simulink model "rd3_mimo_sim_max"  (R2017b)
settings: Solver=ode23tb  StartTime=0.0  StopTime=tsim  FixedStep=0.001  RelTol=1e-3
values from neighbouring files (symbols this model uses):
  a20 = 1    [SISO_Example.m]
  a21 = 2    [SISO_Example.m]
  a22 = 1    [SISO_Example.m]
  Aa = [A,zeros(length(A),length(index_output)) ... (first row only)    [SimVFA.m]
  Aa_M = zeros([12,12,length(TP.etasweep)])    [SimVFA.m]
  Ba = [B; zeros(length(index_output),num_input)]    [SimVFA.m]
  Ba32_aug_M = zeros([12,3,length(TP.etasweep)])    [SimVFA.m]
  Ba32_M = zeros([12,2,length(TP.etasweep)])    [SimVFA.m]
  Ba3_aug_M = zeros([12,3,length(TP.etasweep)])    [SimVFA.m]
  Ba3_M = zeros([12,2,length(TP.etasweep)])    [SimVFA.m]
  Bp = B_c_hold(:,:,SO.eta_nom+1)    [SimVFA.m]
  Ca = [C, zeros(size(C,1),length(index_output)) ... (first row only)    [SimVFA.m]
  Cz = [0,0,0,0,1,0,0,0,0,0 ... (first row only)    [SimVFA.m]
  Kr_M = zeros([2,12,length(TP.etasweep)])    [SimVFA.m]
  Las = Uinv*Lis    [SimVFA.m]
  Las_M = zeros([12,3,length(TP.etasweep)])    [SimVFA.m]
  Ras_M = zeros([3,3,length(TP.etasweep)])    [SimVFA.m]
  Sas1_M = zeros([2,3,length(TP.etasweep)])    [SimVFA.m]
  Sas_M = zeros([3,3,length(TP.etasweep)])    [SimVFA.m]
undefined symbols (not defined in the file or in its folder): Aact, Acmd, Ada_Flag, ahold, Apsim, Bact, Bact_x, Bcmd, Bm, Cact, Cact_dot, Caz, Ccmd, Ccmd_dot, Cm, d00, d10, d11, d20, d21, d22, d_sam, data, Dz, Gamma_l, Gamma_p1, Gamma_p2, Gamma_p3, Gamma_p31, Gamma_p31xm, Gamma_p32, Gamma_vl, i_input_sel, i_state_sel, initstate, input_hold, inputselect, lambda_0, Lambda_s, mu_lambda, mu_psi1, mu_psi2, mu_psi3, mu_psi31, mu_psi32, n_sam, psi1_0, psi2_0, psi31_0, psi31xm_0, psi32_0, psi3_0, samplet, Si1, Si3, state_hold, vlambda_0, x_red_est_0
libraries: simulink x6
(part 1 of 2)
settings Model: SimulationMode=accelerator  Creator=Travis  LastModifiedBy=ben
settings DataIOCC: LimitDataPoints=on  SaveFormat=Structure  SignalLoggingSaveFormat=ModelDataLogs  SaveOutput=off  SignalLogging=off  DSMLogging=off  SaveTime=off  ReturnWorkspaceOutputs=on
settings OptimizationCC: BlockReduction=off  DefaultParameterBehavior=Inlined  BufferReuse=off  ExpressionDepthLimit=2147483647  InitFltsAndDblsToZero=on  LifeSpan=inf
settings DebuggingCC: SaveWithParameterizedLinksMsg=none  UnderspecifiedInitializationDetection=Classic  MergeDetectMultiDrivingBlocksExec=none  SignalResolutionControl=TryResolveAllWithWarning  SolverPrmCheckMsg=warning  MultiTaskDSMMsg=warning  MultiTaskCondExecSysMsg=none  FcnCallInpInsideContextMsg=warning  StateNameClashWarn=warning  StrictBusMsg=Warning  SFUnexpectedBacktrackingDiag=warning  SFNoUnconditionalDefaultTransitionDiag=warning  SFExecutionAtInitializationDiag=none
settings HardwareCC: ProdBitPerPointer=32  ProdBitPerSizeT=32  ProdBitPerPtrDiffT=32  ProdLargestAtomicFloat=None  ProdIntDivRoundTo=Undefined  ProdEndianess=Unspecified  ProdWordSize=32  ProdHWDeviceType=32-bit Generic
settings ModelReferenceCC: PropagateSignalLabelsOutOfModel=off
settings CodeAppCC: StateflowObjectComments=on
settings GRTTargetCC: TargetFcnLib=ansi_tfl_tmw.mat  TargetLangStandard=C89/C90 (ANSI)  GeneratePreprocessorConditionals=Disable all  CombineOutputUpdateFcns=off  GRTInterface=on
settings ConfigComp: CovMetricSettings=dw  CovHtmlReporting=on  CovSaveCumulativeToWorkspaceVar=on  CovSaveSingleToWorkspaceVar=on  CovExternalEMLEnable=off

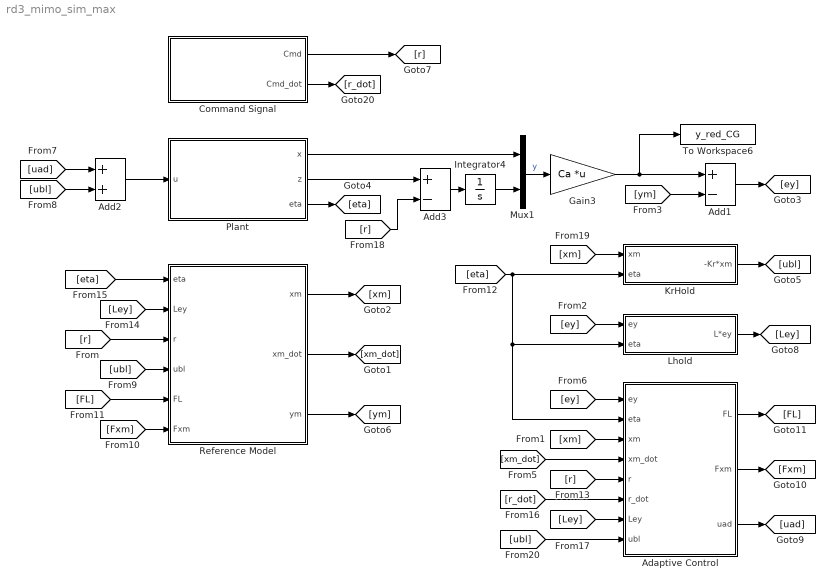
== system rd3_mimo_sim_max ==
  Adaptive Control : Subsystem
  Add1 : Sum  Inputs=+-
  Add2 : Sum
  Add3 : Sum  Inputs=+-
  Command Signal : Subsystem
  Gain3 : Gain  Gain=Ca  Multiplication=Matrix(K*u)
  Integrator4 : Integrator
  KrHold : Subsystem
  Lhold : Subsystem
  Mux1 : Mux  Inputs=2
  Plant : Subsystem
  Reference Model : Subsystem
  To Workspace6 : ToWorkspace  VariableName=y_red_CG  SampleTime=-1
      settings: Decimation=data_deci
  wires:
  Command Signal/1(Cmd) -> [r]
  [ey] -> Lhold/1(ey)
  Lhold/1(L*ey) -> [Ley]
  Mux1/1 -> Gain3/1  "y"
  Command Signal/2(Cmd_dot) -> [r_dot]
  [ym] -> Add1/2
  Add1/1 -> [ey]
  [uad] -> Add2/1
  [ubl] -> Add2/2
  [ey] -> Adaptive Control/1(ey)
  Adaptive Control/1(FL) -> [FL]
  Adaptive Control/2(Fxm) -> [Fxm]
  Adaptive Control/3(uad) -> [uad]
  [eta] -> Lhold/2(eta), Adaptive Control/2(eta), KrHold/2(eta)
  [eta] -> Reference Model/1(eta)
  [Ley] -> Reference Model/2(Ley)
  [r] -> Reference Model/3(r)
  [ubl] -> Reference Model/4(ubl)
  [FL] -> Reference Model/5(FL)
  [Fxm] -> Reference Model/6(Fxm)
  Reference Model/1(xm) -> [xm]
  Reference Model/2(xm_dot) -> [xm_dot]
  Integrator4/1 -> Mux1/2
  Add2/1 -> Plant/1(u)
  Plant/1(x) -> Mux1/1
  Add3/1 -> Integrator4/1
  Plant/2(z) -> Add3/1
  [r] -> Add3/2
  KrHold/1(-Kr*xm) -> [ubl]
  [xm] -> KrHold/1(xm)
  Reference Model/3(ym) -> [ym]
  Gain3/1 -> To Workspace6/1, Add1/1
  [xm] -> Adaptive Control/3(xm)
  [xm_dot] -> Adaptive Control/4(xm_dot)
  [r] -> Adaptive Control/5(r)
  [r_dot] -> Adaptive Control/6(r_dot)
  [Ley] -> Adaptive Control/7(Ley)
  [ubl] -> Adaptive Control/8(ubl)
  Plant/3(eta) -> [eta]

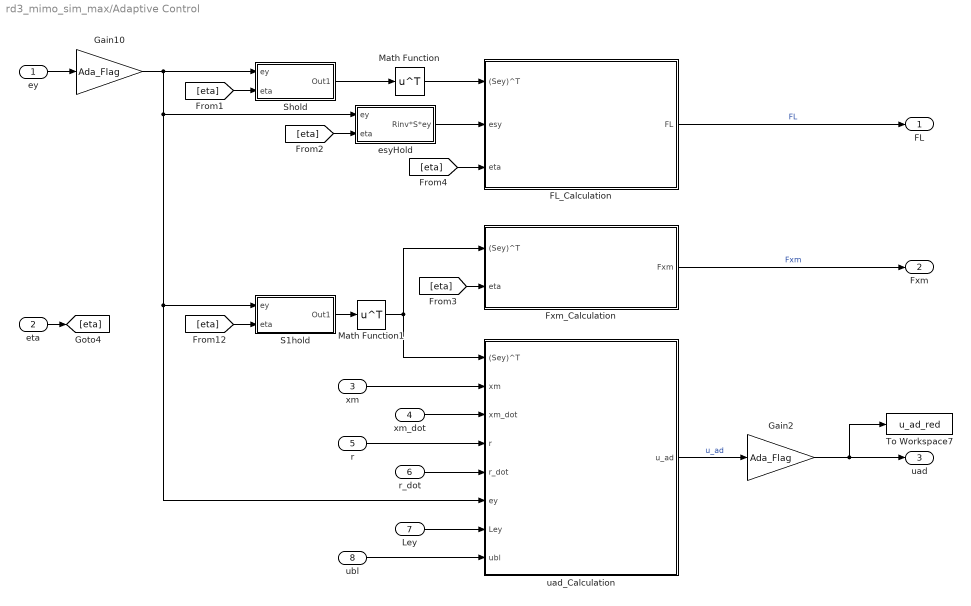
== system rd3_mimo_sim_max/Adaptive Control ==
  ey : Inport
  eta : Inport  Port=2
  xm : Inport  Port=3
  xm_dot : Inport  Port=4
  r : Inport  Port=5
  r_dot : Inport  Port=6
  Ley : Inport  Port=7
  ubl : Inport  Port=8
  FL_Calculation : Subsystem
  Fxm_Calculation : Subsystem
  Gain10 : Gain  Gain=Ada_Flag
  Gain2 : Gain  Gain=Ada_Flag
  Math Function : Math  Operator=transpose  SaturateOnIntegerOverflow=on
  Math Function1 : Math  Operator=transpose  SaturateOnIntegerOverflow=on
  S1hold : Subsystem
  Shold : Subsystem
  To Workspace7 : ToWorkspace  VariableName=u_ad_red  SampleTime=-1
      settings: Decimation=data_deci
  esyHold : Subsystem
  uad_Calculation : Subsystem
  FL : Outport
  Fxm : Outport  Port=2
  uad : Outport  Port=3
  wires:
  Shold/1(Out1) -> Math Function/1
  Math Function/1 -> FL_Calculation/1((Sey)^T)
  S1hold/1(Out1) -> Math Function1/1
  Math Function1/1 -> uad_Calculation/1((Sey)^T), Fxm_Calculation/1((Sey)^T)
  Gain10/1 -> Shold/1(ey), esyHold/1(ey), S1hold/1(ey), uad_Calculation/6(ey)
  uad_Calculation/1(u_ad) -> Gain2/1  "u_ad"
  ey/1 -> Gain10/1
  Fxm_Calculation/1(Fxm) -> Fxm/1  "Fxm"
  FL_Calculation/1(FL) -> FL/1  "FL"
  Gain2/1 -> To Workspace7/1, uad/1
  xm/1 -> uad_Calculation/2(xm)
  xm_dot/1 -> uad_Calculation/3(xm_dot)
  r/1 -> uad_Calculation/4(r)
  r_dot/1 -> uad_Calculation/5(r_dot)
  Ley/1 -> uad_Calculation/7(Ley)
  ubl/1 -> uad_Calculation/8(ubl)
  esyHold/1(Rinv*S*ey) -> FL_Calculation/2(esy)
  eta/1 -> [eta]
  [eta] -> S1hold/2(eta)
  [eta] -> Shold/2(eta)
  [eta] -> esyHold/2(eta)
  [eta] -> Fxm_Calculation/2(eta)
  [eta] -> FL_Calculation/3(eta)

== system rd3_mimo_sim_max/Command Signal ==
  Clock : Clock
  Filter : Subsystem
  From Workspace : FromWorkspace  VariableName=r_timeseries  SampleTime=0  Interpolate=off  OutputAfterFinalValue=Holding final value
  To Workspace14 : ToWorkspace  VariableName=r_cmd  SampleTime=-1
      settings: Decimation=data_deci
  To Workspace6 : ToWorkspace  VariableName=t_sim  SampleTime=-1
      settings: Decimation=data_deci
  Cmd : Outport
  Cmd_dot : Outport  Port=2
  wires:
  Clock/1 -> To Workspace6/1
  Filter/1(Cmd) -> To Workspace14/1, Cmd/1
  Filter/2(Cmd_dot) -> Cmd_dot/1
  From Workspace/1 -> Filter/1(r)

== system rd3_mimo_sim_max/KrHold ==
  xm : Inport
  eta : Inport  Port=2
  Constant2 : Constant  Value=Kr_M
  Gain : Gain  Gain=180/pi
  Gain18 : Gain  Gain=-1
  Matrix Multiply6 : Product  Multiplication=Matrix(*)
  Subsystem1 : Subsystem
      mask Display: disp('matrix-interp');
  To Workspace8 : ToWorkspace  VariableName=u_bl_red  SampleTime=-1
      settings: Decimation=data_deci
  -Kr*xm : Outport
  wires:
  eta/1 -> Gain/1
  Gain/1 -> Subsystem1/1(In1)
  Subsystem1/1(Out1) -> Matrix Multiply6/1
  xm/1 -> Matrix Multiply6/2
  Constant2/1 -> Subsystem1/2(In2)
  Gain18/1 -> -Kr*xm/1, To Workspace8/1  "u_bl"
  Matrix Multiply6/1 -> Gain18/1

== system rd3_mimo_sim_max/Lhold ==
  ey : Inport
  eta : Inport  Port=2
  Constant2 : Constant  Value=Las_M
  Gain : Gain  Gain=180/pi
  Matrix Multiply6 : Product  Multiplication=Matrix(*)
  Subsystem1 : Subsystem
      mask Display: disp('matrix-interp');
  L*ey : Outport
  wires:
  eta/1 -> Gain/1
  Subsystem1/1(Out1) -> Matrix Multiply6/1
  ey/1 -> Matrix Multiply6/2
  Matrix Multiply6/1 -> L*ey/1
  Gain/1 -> Subsystem1/1(In1)
  Constant2/1 -> Subsystem1/2(In2)

== system rd3_mimo_sim_max/Plant ==
  u : Inport
  Actuators : Subsystem
  Add : Sum  Inputs=3
  Add1 : Sum  Inputs=2
  Gain1 : Gain  Gain=Dz  Multiplication=Matrix(K*u)
  Gain24 : Gain  Gain=Lambda_s  Multiplication=Matrix(K*u)
  Gain5 : Gain  Gain=inputselect  Multiplication=Matrix(K*u)
  Gain9 : Gain  Gain=Cz  Multiplication=Matrix(K*u)
  Mux2 : Mux  Inputs=2
  Noise : simulink/Sources/Band-Limited White Noise  Cov=n_mean  Ts=n_sam  seed=n_seed
  Noise1 : simulink/Sources/Band-Limited White Noise  Cov=d_mean  Ts=d_sam  seed=d_seed
  NonLinear VFA Model : Subsystem
  To Workspace1 : ToWorkspace  VariableName=x_red  SampleTime=-1
      settings: Decimation=data_deci
  To Workspace12 : ToWorkspace  VariableName=z_red  SampleTime=-1
      settings: Decimation=data_deci
  Wind Gust Model : Subsystem
  x : Outport
  z : Outport  Port=2
  eta : Outport  Port=3
  wires:
  Mux2/1 -> x/1, Gain9/1
  NonLinear VFA Model/2(States Rel. to Trim) -> Mux2/1, Actuators/2(coupled)
  Gain1/1 -> Add/2
  Gain9/1 -> Add/1
  Actuators/2(States) -> Mux2/2
  Add/1 -> To Workspace12/1, z/1  "Plant"
  Gain5/1 -> NonLinear VFA Model/1(Controls)
  NonLinear VFA Model/1(States) -> To Workspace1/1
  Wind Gust Model/1(Gust) -> NonLinear VFA Model/2(Gust)
  Gain24/1 -> Gain1/1, Actuators/1(Comand)
  Noise/1 -> Add/3
  Noise1/1 -> Add1/1
  Actuators/1(Control) -> Add1/2
  Add1/1 -> Gain5/1
  u/1 -> Gain24/1
  NonLinear VFA Model/3(eta) -> eta/1

== system rd3_mimo_sim_max/Reference Model ==
  eta : Inport
  Ley : Inport  Port=2
  r : Inport  Port=3
  ubl : Inport  Port=4
  FL : Inport  Port=5
  Fxm : Inport  Port=6
  Add3 : Sum  Inputs=+++++-
  Ahold : Subsystem
  Gain16 : Gain  Gain=Ba  Multiplication=Matrix(K*u)
  Gain21 : Gain  Gain=Bm  Multiplication=Matrix(K*u)
  Gain22 : Gain  Gain=Caz  Multiplication=Matrix(K*u)
  Gain8 : Gain  Gain=Cm  Multiplication=Matrix(K*u)
  Integrator1 : Integrator  InitialCondition=x_red_est_0
  To Workspace11 : ToWorkspace  VariableName=z_red_est  SampleTime=-1
      settings: Decimation=data_deci
  To Workspace3 : ToWorkspace  VariableName=x_red_est  SampleTime=-1
      settings: Decimation=data_deci
  To Workspace5 : ToWorkspace  VariableName=y_red_est_CG  SampleTime=-1
      settings: Decimation=data_deci
  xm : Outport
  xm_dot : Outport  Port=2
  ym : Outport  Port=3
  wires:
  Gain21/1 -> Add3/3
  Ahold/1(Out1) -> Add3/1
  Add3/1 -> xm_dot/1, Integrator1/1
  eta/1 -> Ahold/2(eta)
  r/1 -> Gain21/1
  ubl/1 -> Gain16/1
  Gain16/1 -> Add3/4
  Integrator1/1 -> To Workspace3/1, Ahold/1(State), Gain22/1, Gain8/1, xm/1  "xm"
  Fxm/1 -> Add3/6
  FL/1 -> Add3/5
  Ley/1 -> Add3/2
  Gain22/1 -> To Workspace11/1  "Ref"
  Gain8/1 -> ym/1, To Workspace5/1  "ym"

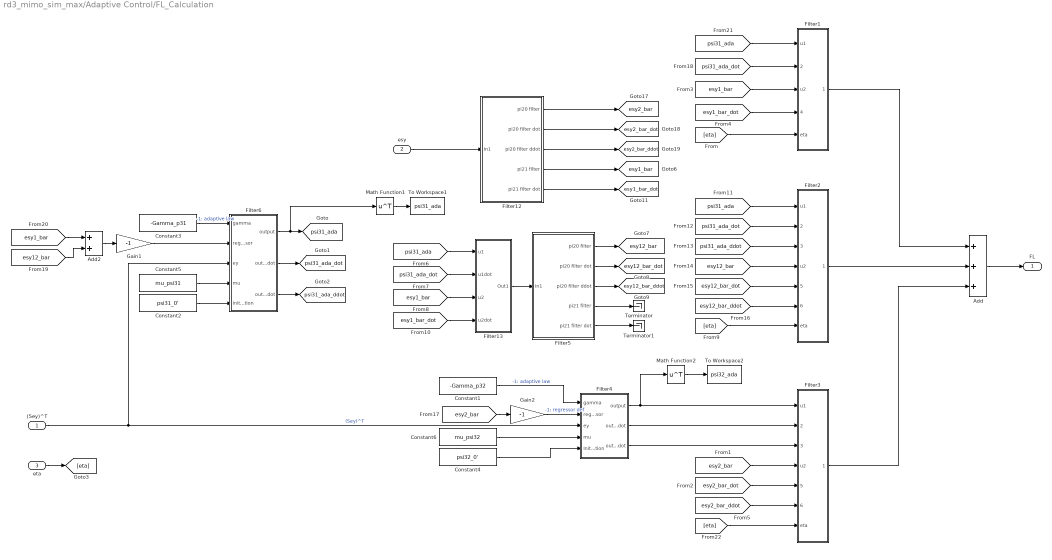
== system rd3_mimo_sim_max/Adaptive Control/FL_Calculation ==
  (Sey)^T : Inport
  esy : Inport  Port=2
  eta : Inport  Port=3
  Add : Sum  Inputs=3
  Add2 : Sum
  Constant1 : Constant  Value=-Gamma_p32  VectorParams1D=off
  Constant2 : Constant  Value=psi31_0'  VectorParams1D=off
  Constant3 : Constant  Value=-Gamma_p31  VectorParams1D=off
  Constant4 : Constant  Value=psi32_0'  VectorParams1D=off
  Constant5 : Constant  Value=mu_psi31  VectorParams1D=off
  Constant6 : Constant  Value=mu_psi32  VectorParams1D=off
  Filter1 : Subsystem
      mask Display: disp('F32')
  Filter12 : Subsystem
      mask Display: disp('pi20 and pi21 filter')
  Filter13 : Subsystem
      mask Display: disp('D1 Mixer')
  Filter2 : Subsystem
      mask Display: disp('F33')
  Filter3 : Subsystem
      mask Display: disp('F33')
  Filter4 : Subsystem
      mask Display: disp('2nd order Tuner')
  Filter5 : Subsystem
      mask Display: disp('pi20 and pi21 filter')
  Filter6 : Subsystem
      mask Display: disp('2nd order Tuner')
  Gain1 : Gain  Gain=-1
  Gain2 : Gain  Gain=-1
  Math Function1 : Math  Operator=transpose  SaturateOnIntegerOverflow=on
  Math Function2 : Math  Operator=transpose  SaturateOnIntegerOverflow=on
  Terminator : Terminator
  Terminator1 : Terminator
  To Workspace1 : ToWorkspace  VariableName=psi31_ada  SampleTime=-1
      settings: Decimation=data_deci
  To Workspace2 : ToWorkspace  VariableName=psi32_ada  SampleTime=-1
      settings: Decimation=data_deci
  FL : Outport
  tag scope: esy12_bar=global, esy12_bar_ddot=global, esy12_bar_dot=global, esy1_bar=global, esy1_bar_dot=global, esy2_bar=global, esy2_bar_ddot=global, esy2_bar_dot=global, psi31_ada=global, psi31_ada_ddot=global, psi31_ada_dot=global
  wires:
  (Sey)^T/1 -> Filter6/3(ey), Filter4/3(ey)  "(Sey)^T"
  Constant3/1 -> Filter6/1(gamma)  "-1: adaptive law"
  Add2/1 -> Gain1/1
  [esy1_bar_dot] -> Filter1/4(u2dot)
  [esy1_bar] -> Filter1/3(u2)
  Filter6/1(output) -> Math Function1/1, [psi31_ada]
  Filter6/2(output_dot) -> [psi31_ada_dot]
  Filter6/3(output_ddot) -> [psi31_ada_ddot]
  Add/1 -> FL/1
  Filter1/1(Out1) -> Add/1
  Math Function1/1 -> To Workspace1/1
  Constant1/1 -> Filter4/1(gamma)  "-1: adaptive law"
  Gain2/1 -> Filter4/2(regressor)  "-1: regressor def"
  Filter4/2(output_dot) -> Filter3/2(u1dot)
  Filter4/3(output_ddot) -> Filter3/3(u1ddot)
  Filter4/1(output) -> Math Function2/1, Filter3/1(u1)
  Math Function2/1 -> To Workspace2/1
  esy/1 -> Filter12/1(In1)
  Filter12/4(pi21 filter) -> [esy1_bar]
  Filter12/5(pi21 filter dot) -> [esy1_bar_dot]
  Filter12/1(pi20 filter) -> [esy2_bar]
  Filter12/2(pi20 filter dot) -> [esy2_bar_dot]
  Filter12/3(pi20 filter ddot) -> [esy2_bar_ddot]
  [esy2_bar] -> Filter3/4(u2)
  [esy2_bar_dot] -> Filter3/5(u2dot)
  [esy2_bar_ddot] -> Filter3/6(u2ddot)
  Filter3/1(Out1) -> Add/3
  [psi31_ada] -> Filter13/1(u1)
  [psi31_ada_dot] -> Filter13/2(u1dot)
  [esy1_bar] -> Filter13/3(u2)
  [esy1_bar_dot] -> Filter13/4(u2dot)
  Filter13/1(Out1) -> Filter5/1(In1)
  Filter5/4(pi21 filter) -> Terminator/1
  Filter5/5(pi21 filter dot) -> Terminator1/1
  Filter5/1(pi20 filter) -> [esy12_bar]
  Filter5/2(pi20 filter dot) -> [esy12_bar_dot]
  Filter5/3(pi20 filter ddot) -> [esy12_bar_ddot]
  [psi31_ada] -> Filter2/1(u1)
  [psi31_ada_dot] -> Filter2/2(u1dot)
  [psi31_ada_ddot] -> Filter2/3(u1ddot)
  [esy12_bar] -> Filter2/4(u2)
  [esy12_bar_dot] -> Filter2/5(u2dot)
  [esy12_bar_ddot] -> Filter2/6(u2ddot)
  Filter2/1(Out1) -> Add/2
  [esy2_bar] -> Gain2/1
  [esy12_bar] -> Add2/2
  [esy1_bar] -> Add2/1
  Constant2/1 -> Filter6/5(InitialCondition)
  Constant4/1 -> Filter4/5(InitialCondition)
  Constant5/1 -> Filter6/4(mu)
  Constant6/1 -> Filter4/4(mu)
  Gain1/1 -> Filter6/2(regressor)
  [psi31_ada_dot] -> Filter1/2(u1dot)
  [psi31_ada] -> Filter1/1(u1)
  eta/1 -> [eta]
  [eta] -> Filter1/5(eta)
  [eta] -> Filter2/7(eta)
  [eta] -> Filter3/7(eta)

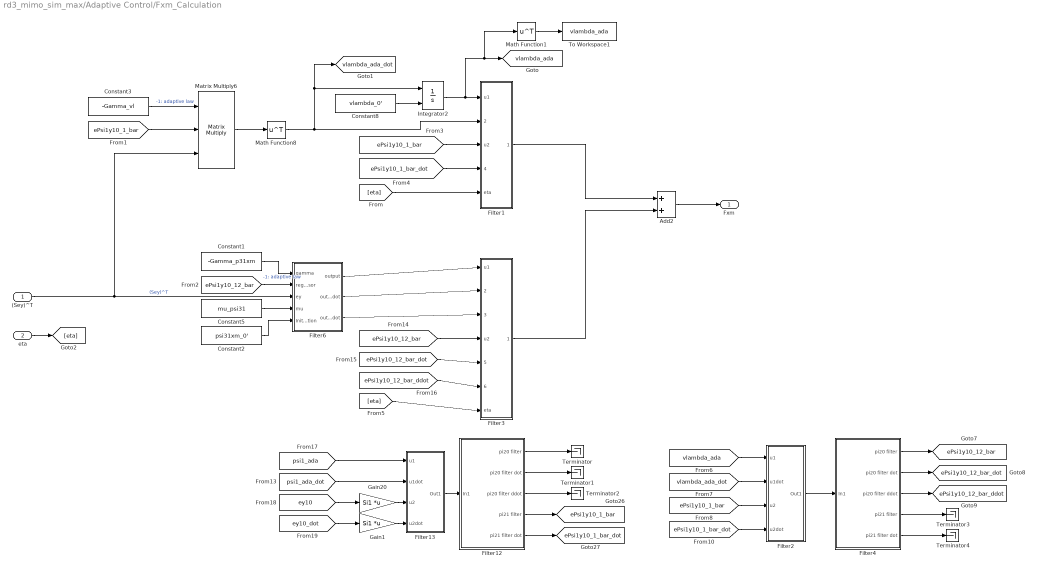
== system rd3_mimo_sim_max/Adaptive Control/Fxm_Calculation ==
  (Sey)^T : Inport
  eta : Inport  Port=2
  Add2 : Sum
  Constant1 : Constant  Value=-Gamma_p31xm  VectorParams1D=off
  Constant2 : Constant  Value=psi31xm_0'  VectorParams1D=off
  Constant3 : Constant  Value=-Gamma_vl  VectorParams1D=off
  Constant5 : Constant  Value=mu_psi31  VectorParams1D=off
  Constant8 : Constant  Value=vlambda_0'  VectorParams1D=off
  Filter1 : Subsystem
      mask Display: disp('F32')
  Filter12 : Subsystem
      mask Display: disp('pi20 and pi21 filter')
  Filter13 : Subsystem
      mask Display: disp('D1 Mixer')
  Filter2 : Subsystem
      mask Display: disp('D1 Mixer')
  Filter3 : Subsystem
      mask Display: disp('F33')
  Filter4 : Subsystem
      mask Display: disp('pi20 and pi21 filter')
  Filter6 : Subsystem
      mask Display: disp('2nd order Tuner')
  Gain1 : Gain  Gain=Si1  Multiplication=Matrix(K*u)
  Gain20 : Gain  Gain=Si1  Multiplication=Matrix(K*u)
  Integrator2 : Integrator  InitialConditionSource=external  InitialCondition=lambda_0'
  Math Function1 : Math  Operator=transpose  SaturateOnIntegerOverflow=on
  Math Function8 : Math  Operator=transpose  SaturateOnIntegerOverflow=on
  Matrix Multiply6 : Product  Inputs=3  Multiplication=Matrix(*)
  Terminator{,1..4} (5 alike) : Terminator
  To Workspace1 : ToWorkspace  VariableName=vlambda_ada  SampleTime=-1
      settings: Decimation=data_deci
  Fxm : Outport
  tag scope: ePsi1y10_12_bar=global, ePsi1y10_12_bar_ddot=global, ePsi1y10_12_bar_dot=global, ePsi1y10_1_bar=global, ePsi1y10_1_bar_dot=global, vlambda_ada=global, vlambda_ada_dot=global
  wires:
  Filter13/1(Out1) -> Filter12/1(In1)
  Filter12/1(pi20 filter) -> Terminator/1
  Filter12/2(pi20 filter dot) -> Terminator1/1
  Filter12/3(pi20 filter ddot) -> Terminator2/1
  [psi1_ada_dot] -> Filter13/2(u1dot)
  [psi1_ada] -> Filter13/1(u1)
  [ey10] -> Gain20/1
  [ey10_dot] -> Gain1/1
  Filter12/4(pi21 filter) -> [ePsi1y10_1_bar]
  Filter12/5(pi21 filter dot) -> [ePsi1y10_1_bar_dot]
  (Sey)^T/1 -> Matrix Multiply6/3, Filter6/3(ey)  "(Sey)^T"
  Constant3/1 -> Matrix Multiply6/1  "-1: adaptive law"
  [ePsi1y10_1_bar] -> Matrix Multiply6/2
  [ePsi1y10_1_bar_dot] -> Filter1/4(u2dot)
  [ePsi1y10_1_bar] -> Filter1/3(u2)
  Integrator2/1 -> Filter1/1(u1), Math Function1/1, [vlambda_ada]
  Math Function8/1 -> [vlambda_ada_dot], Integrator2/1, Filter1/2(u1dot)
  Math Function1/1 -> To Workspace1/1
  [vlambda_ada] -> Filter2/1(u1)
  [vlambda_ada_dot] -> Filter2/2(u1dot)
  [ePsi1y10_1_bar] -> Filter2/3(u2)
  [ePsi1y10_1_bar_dot] -> Filter2/4(u2dot)
  Filter2/1(Out1) -> Filter4/1(In1)
  Filter4/4(pi21 filter) -> Terminator3/1
  Filter4/5(pi21 filter dot) -> Terminator4/1
  Filter4/1(pi20 filter) -> [ePsi1y10_12_bar]
  Filter4/2(pi20 filter dot) -> [ePsi1y10_12_bar_dot]
  Filter4/3(pi20 filter ddot) -> [ePsi1y10_12_bar_ddot]
  [ePsi1y10_12_bar] -> Filter3/4(u2)
  [ePsi1y10_12_bar_dot] -> Filter3/5(u2dot)
  [ePsi1y10_12_bar_ddot] -> Filter3/6(u2ddot)
  Add2/1 -> Fxm/1
  Gain20/1 -> Filter13/3(u2)
  Gain1/1 -> Filter13/4(u2dot)
  Filter6/1(output) -> Filter3/1(u1)
  Filter6/2(output_dot) -> Filter3/2(u1dot)
  Filter6/3(output_ddot) -> Filter3/3(u1ddot)
  Matrix Multiply6/1 -> Math Function8/1
  Constant2/1 -> Filter6/5(InitialCondition)
  Constant5/1 -> Filter6/4(mu)
  Constant8/1 -> Integrator2/2
  Constant1/1 -> Filter6/1(gamma)  "-1: adaptive law"
  [ePsi1y10_12_bar] -> Filter6/2(regressor)
  Filter1/1(Out1) -> Add2/1
  Filter3/1(Out1) -> Add2/2
  eta/1 -> [eta]
  [eta] -> Filter1/5(eta)
  [eta] -> Filter3/7(eta)

== system rd3_mimo_sim_max/Adaptive Control/S1hold ==
  ey : Inport
  eta : Inport  Port=2
  Constant2 : Constant  Value=Sas1_M
  Gain : Gain  Gain=180/pi
  Matrix Multiply6 : Product  Multiplication=Matrix(*)
  Subsystem1 : Subsystem
      mask Display: disp('matrix-interp');
  Out1 : Outport
  wires:
  eta/1 -> Gain/1
  ey/1 -> Matrix Multiply6/2
  Matrix Multiply6/1 -> Out1/1
  Gain/1 -> Subsystem1/1(In1)
  Constant2/1 -> Subsystem1/2(In2)
  Subsystem1/1(Out1) -> Matrix Multiply6/1

== system rd3_mimo_sim_max/Adaptive Control/Shold ==
  ey : Inport
  eta : Inport  Port=2
  Constant2 : Constant  Value=Sas_M
  Gain : Gain  Gain=180/pi
  Matrix Multiply6 : Product  Multiplication=Matrix(*)
  Subsystem1 : Subsystem
      mask Display: disp('matrix-interp');
  Out1 : Outport
  wires:
  eta/1 -> Gain/1
  Subsystem1/1(Out1) -> Matrix Multiply6/1
  ey/1 -> Matrix Multiply6/2
  Matrix Multiply6/1 -> Out1/1
  Gain/1 -> Subsystem1/1(In1)
  Constant2/1 -> Subsystem1/2(In2)

== system rd3_mimo_sim_max/Adaptive Control/esyHold ==
  ey : Inport
  eta : Inport  Port=2
  Constant1 : Constant  Value=Sas_M
  Constant2 : Constant  Value=Ras_M
  Gain : Gain  Gain=180/pi
  Gain1 : Gain  Gain=180/pi
  Matrix Multiply6 : Product  Inputs=3  Multiplication=Matrix(*)
  Subsystem1 : Subsystem
      mask Display: disp('matrix-interp');
  Subsystem2 : Subsystem
      mask Display: disp('matrix-interp');
  Rinv*S*ey : Outport
  wires:
  Subsystem1/1(Out1) -> Matrix Multiply6/1
  ey/1 -> Matrix Multiply6/3
  Matrix Multiply6/1 -> Rinv*S*ey/1
  Subsystem2/1(Out1) -> Matrix Multiply6/2
  Gain/1 -> Subsystem1/1(In1)
  Constant2/1 -> Subsystem1/2(In2)
  Gain1/1 -> Subsystem2/1(In1)
  Constant1/1 -> Subsystem2/2(In2)
  eta/1 -> Gain1/1, Gain/1

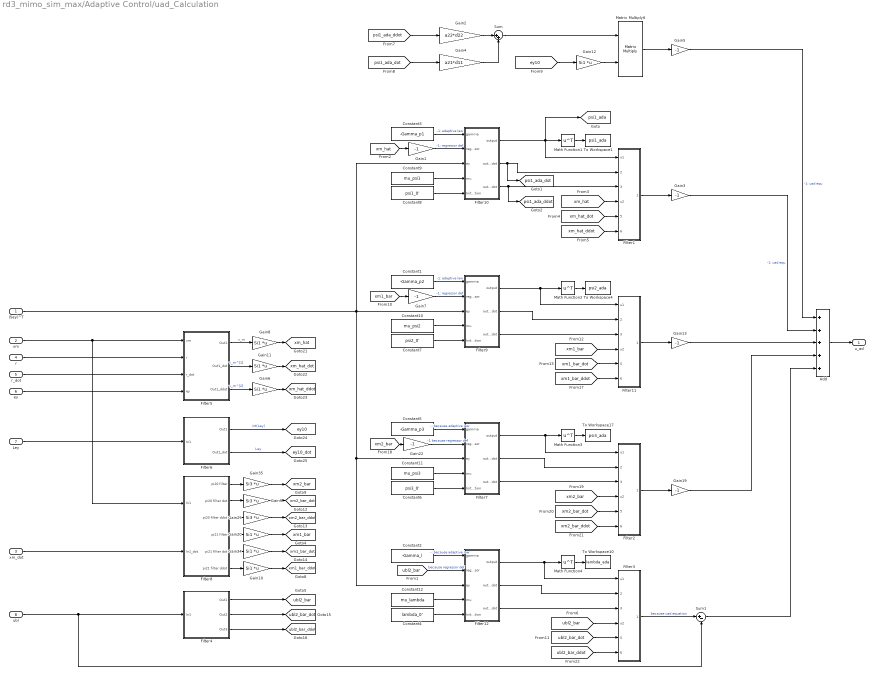
== system rd3_mimo_sim_max/Adaptive Control/uad_Calculation ==
  (Sey)^T : Inport
  xm : Inport  Port=2
  xm_dot : Inport  Port=3
  r : Inport  Port=4
  r_dot : Inport  Port=5
  ey : Inport  Port=6
  Ley : Inport  Port=7
  ubl : Inport  Port=8
  Add : Sum  Inputs=5
  Constant1 : Constant  Value=-Gamma_p2  VectorParams1D=off
  Constant10 : Constant  Value=mu_psi2  VectorParams1D=off
  Constant11 : Constant  Value=mu_psi3  VectorParams1D=off
  Constant12 : Constant  Value=mu_lambda  VectorParams1D=off
  Constant2 : Constant  Value=-Gamma_l  VectorParams1D=off
  Constant3 : Constant  Value=-Gamma_p1  VectorParams1D=off
  Constant4 : Constant  Value=lambda_0'  VectorParams1D=off
  Constant5 : Constant  Value=-Gamma_p3  VectorParams1D=off
  Constant6 : Constant  Value=psi3_0'  VectorParams1D=off
  Constant7 : Constant  Value=psi2_0'  VectorParams1D=off
  Constant8 : Constant  Value=psi1_0'  VectorParams1D=off
  Constant9 : Constant  Value=mu_psi1  VectorParams1D=off
  Filter1 : Subsystem
      mask Display: disp('pi22 Mixer')
  Filter10 : Subsystem
      mask Display: disp('2nd order Tuner')
  Filter11 : Subsystem
      mask Display: disp('pi22 Mixer')
  Filter12 : Subsystem
      mask Display: disp('2nd order Tuner')
  Filter2 : Subsystem
      mask Display: disp('pi22 Mixer')
  Filter3 : Subsystem
      mask Display: disp('pi22 Mixer')
  Filter4 : Subsystem
      mask Display: disp('pi20/a22 filter')
  Filter5 : Subsystem
      mask Display: disp('pseudo filter 1')
  Filter6 : Subsystem
      mask Display: disp('ePsiy filter')
  Filter7 : Subsystem
      mask Display: disp('2nd order Tuner')
  Filter8 : Subsystem
      mask Display: disp('pi20 and pi21 mix filter')
  Filter9 : Subsystem
      mask Display: disp('2nd order Tuner')
  Gain{1,3,5,7,13,19,22} (7 alike) : Gain  Gain=-1
  Gain{6,8,10..12,20,34} (7 alike) : Gain  Gain=Si1  Multiplication=Matrix(K*u)
  Gain2 : Gain  Gain=a22*d22
  Gain29 : Gain  Gain=Si3  Multiplication=Matrix(K*u)
  Gain35 : Gain  Gain=Si3  Multiplication=Matrix(K*u)
  Gain4 : Gain  Gain=a21*d11
  Gain9 : Gain  Gain=Si3  Multiplication=Matrix(K*u)
  Math Function{1..4} (4 alike) : Math  Operator=transpose  SaturateOnIntegerOverflow=on
  Matrix Multiply6 : Product  Multiplication=Matrix(*)
  Sum : Sum  Inputs=|++
  Sum1 : Sum  Inputs=|+-
  To Workspace1 : ToWorkspace  VariableName=psi1_ada  SampleTime=-1
      settings: Decimation=data_deci
  To Workspace10 : ToWorkspace  VariableName=lambda_ada  SampleTime=-1
      settings: Decimation=data_deci
  To Workspace17 : ToWorkspace  VariableName=psi3_ada  SampleTime=-1
      settings: Decimation=data_deci
  To Workspace4 : ToWorkspace  VariableName=psi2_ada  SampleTime=-1
      settings: Decimation=data_deci
  u_ad : Outport
  tag scope: ey10=global, ey10_dot=global, psi1_ada=global, psi1_ada_ddot=global, psi1_ada_dot=global, ubl2_bar=global, ubl2_bar_ddot=global, ubl2_bar_dot=global, xm1_bar=global, xm1_bar_ddot=global, xm1_bar_dot=global, xm2_bar=global, xm2_bar_ddot=global, xm2_bar_dot=global, xm_hat=global, xm_hat_ddot=global, xm_hat_dot=global
  wires:
  Constant1/1 -> Filter9/1(gamma)  "-1: adaptive law"
  [xm1_bar] -> Gain7/1
  Gain7/1 -> Filter9/2(regressor)  "-1: regressor def"
  Filter9/1(output) -> Math Function2/1, Filter11/1(u1)
  Filter9/2(output_dot) -> Filter11/2(u1dot)
  Filter9/3(output_ddot) -> Filter11/3(u1ddot)
  [xm1_bar] -> Filter11/4(u2)
  [xm1_bar_dot] -> Filter11/5(u2dot)
  [xm1_bar_ddot] -> Filter11/6(u2ddot)
  Filter11/1(Out1) -> Gain13/1
  Constant5/1 -> Filter7/1(gamma)  "-: because adaptive law"
  [xm2_bar] -> Gain22/1
  Gain22/1 -> Filter7/2(regressor)  "-1 because regressor def"
  Filter7/1(output) -> Filter2/1(u1), Math Function3/1
  Filter7/2(output_dot) -> Filter2/2(u1dot)
  Filter7/3(output_ddot) -> Filter2/3(u1ddot)
  [xm2_bar] -> Filter2/4(u2)
  [xm2_bar_dot] -> Filter2/5(u2dot)
  [xm2_bar_ddot] -> Filter2/6(u2ddot)
  Filter2/1(Out1) -> Gain19/1
  Constant2/1 -> Filter12/1(gamma)  "-: because adaptive law"
  [ubl2_bar] -> Filter12/2(regressor)  "because regressor def"
  Filter12/1(output) -> Math Function4/1, Filter3/1(u1)
  Filter12/2(output_dot) -> Filter3/2(u1dot)
  Filter12/3(output_ddot) -> Filter3/3(u1ddot)
  [ubl2_bar] -> Filter3/4(u2)
  [ubl2_bar_dot] -> Filter3/5(u2dot)
  [ubl2_bar_ddot] -> Filter3/6(u2ddot)
  (Sey)^T/1 -> Filter10/3(ey), Filter9/3(ey), Filter12/3(ey), Filter7/3(ey)
  Gain13/1 -> Add/3
  Gain19/1 -> Add/4
  Constant3/1 -> Filter10/1(gamma)  "-1: adaptive law"
  [xm_hat] -> Gain1/1
  Gain1/1 -> Filter10/2(regressor)  "-1: regressor def"
  [xm_hat_ddot] -> Filter1/6(u2ddot)
  [xm_hat_dot] -> Filter1/5(u2dot)
  [xm_hat] -> Filter1/4(u2)
  Filter10/1(output) -> Filter1/1(u1), [psi1_ada], Math Function1/1
  Filter10/2(output_dot) -> [psi1_ada_dot], Filter1/2(u1dot)
  Filter10/3(output_ddot) -> Filter1/3(u1ddot), [psi1_ada_ddot]
  Filter1/1(Out1) -> Gain3/1
  Add/1 -> u_ad/1
  [psi1_ada_ddot] -> Gain2/1
  Gain3/1 -> Add/2  "-1: uad equ"
  [psi1_ada_dot] -> Gain4/1
  Gain2/1 -> Sum/1
  Gain4/1 -> Sum/2
  Math Function1/1 -> To Workspace1/1
  Math Function2/1 -> To Workspace4/1
  Math Function3/1 -> To Workspace17/1
  Math Function4/1 -> To Workspace10/1
  Sum/1 -> Matrix Multiply6/1
  [ey10] -> Gain12/1
  Matrix Multiply6/1 -> Gain5/1
  Gain5/1 -> Add/1  "-1: uad equ"
  xm/1 -> Filter8/1(In1), Filter5/1(xm)
  ubl/1 -> Sum1/2, Filter4/1(In1)
  Filter4/1(Out1) -> [ubl2_bar]
  Filter8/1(pi20 filter) -> Gain35/1
  Filter8/4(pi21 filter) -> Gain20/1
  Gain20/1 -> [xm1_bar]
  Gain35/1 -> [xm2_bar]
  Filter8/2(pi20 filter dot) -> Gain9/1
  Gain9/1 -> [xm2_bar_dot]
  Filter8/3(pi20 filter ddot) -> Gain29/1
  Gain29/1 -> [xm2_bar_ddot]
  Filter8/5(pi21 filter dot) -> Gain34/1
  Gain34/1 -> [xm1_bar_dot]
  Filter4/3(Out3) -> [ubl2_bar_ddot]
  Filter4/2(Out2) -> [ubl2_bar_dot]
  xm_dot/1 -> Filter8/2(In1_dot)
  Filter8/6(pi21 filter ddot) -> Gain10/1
  Gain10/1 -> [xm1_bar_ddot]
  ey/1 -> Filter5/4(ey)
  Filter5/3(Out1_ddot) -> Gain6/1  "v_m^[2]"
  Filter5/2(Out1_dot) -> Gain11/1  "v_m^[1]"
  Filter5/1(Out1) -> Gain8/1  "v_m"
  Gain8/1 -> [xm_hat]
  Gain11/1 -> [xm_hat_dot]
  Gain6/1 -> [xm_hat_ddot]
  Ley/1 -> Filter6/1(In1)
  Filter6/1(Out1) -> [ey10]  "int(Ley)"
  Filter6/2(Out1_dot) -> [ey10_dot]  "Ley"
  Gain12/1 -> Matrix Multiply6/2
  Constant4/1 -> Filter12/5(InitialCondition)
  Constant6/1 -> Filter7/5(InitialCondition)
  Constant7/1 -> Filter9/5(InitialCondition)
  Constant8/1 -> Filter10/5(InitialCondition)
  Sum1/1 -> Add/5
  Constant9/1 -> Filter10/4(mu)
  Constant10/1 -> Filter9/4(mu)
  Constant11/1 -> Filter7/4(mu)
  Constant12/1 -> Filter12/4(mu)
  r/1 -> Filter5/2(r)
  r_dot/1 -> Filter5/3(r_dot)
  Filter3/1(Out1) -> Sum1/1  "because uad equation"

== system rd3_mimo_sim_max/Command Signal/Filter ==
  r : Inport
  Gain : Gain  Gain=Bcmd  Multiplication=Matrix(K*u)
  Gain1 : Gain  Gain=Acmd  Multiplication=Matrix(K*u)
  Gain2 : Gain  Gain=Ccmd  Multiplication=Matrix(K*u)
  Gain3 : Gain  Gain=Ccmd_dot  Multiplication=Matrix(K*u)
  Integrator : Integrator
  Sum : Sum  Inputs=|++
  Cmd : Outport
  Cmd_dot : Outport  Port=2
  wires:
  r/1 -> Gain/1
  Sum/1 -> Integrator/1
  Integrator/1 -> Gain1/1, Gain3/1, Gain2/1
  Gain/1 -> Sum/1
  Gain1/1 -> Sum/2
  Gain2/1 -> Cmd/1
  Gain3/1 -> Cmd_dot/1

== system rd3_mimo_sim_max/KrHold/Subsystem1 ==
  In1 : Inport
  In2 : Inport  Port=2
  Bias1 : Bias  Bias=1
  Direct Lookup Table (n-D)2 : LookupNDDirect  NumberOfTableDimensions=3  InputsSelectThisObjectFromTable=2-D Matrix  TableIsInput=on  Table=ahold
  Direct Lookup Table (n-D)3 : LookupNDDirect  NumberOfTableDimensions=3  InputsSelectThisObjectFromTable=2-D Matrix  TableIsInput=on  Table=ahold
  Fcn1 : Fcn  Expr=1-u(1)
  Prelookup1 : PreLookup  BreakpointsData=etasweep  ExtrapMethod=Linear
  Product2 : Product  RndMeth=Zero
  Product3 : Product  RndMeth=Zero
  Sum1 : Sum  Inputs=|++
  Out1 : Outport
  wires:
  In1/1 -> Prelookup1/1
  Sum1/1 -> Out1/1
  Prelookup1/1 -> Direct Lookup Table (n-D)3/1, Bias1/1
  Direct Lookup Table (n-D)2/1 -> Product2/1
  Prelookup1/2 -> Product2/2, Fcn1/1
  Direct Lookup Table (n-D)3/1 -> Product3/1
  Product2/1 -> Sum1/1
  Product3/1 -> Sum1/2
  Bias1/1 -> Direct Lookup Table (n-D)2/1
  In2/1 -> Direct Lookup Table (n-D)3/2, Direct Lookup Table (n-D)2/2
  Fcn1/1 -> Product3/2

== system rd3_mimo_sim_max/Lhold/Subsystem1 ==
  In1 : Inport
  In2 : Inport  Port=2
  Bias1 : Bias  Bias=1
  Direct Lookup Table (n-D)2 : LookupNDDirect  NumberOfTableDimensions=3  InputsSelectThisObjectFromTable=2-D Matrix  TableIsInput=on  Table=ahold
  Direct Lookup Table (n-D)3 : LookupNDDirect  NumberOfTableDimensions=3  InputsSelectThisObjectFromTable=2-D Matrix  TableIsInput=on  Table=ahold
  Fcn1 : Fcn  Expr=1-u(1)
  Prelookup1 : PreLookup  BreakpointsData=etasweep  ExtrapMethod=Linear
  Product2 : Product  RndMeth=Zero
  Product3 : Product  RndMeth=Zero
  Sum1 : Sum  Inputs=|++
  Out1 : Outport
  wires:
  In1/1 -> Prelookup1/1
  Sum1/1 -> Out1/1
  Prelookup1/1 -> Direct Lookup Table (n-D)3/1, Bias1/1
  Direct Lookup Table (n-D)2/1 -> Product2/1
  Prelookup1/2 -> Product2/2, Fcn1/1
  Direct Lookup Table (n-D)3/1 -> Product3/1
  Product2/1 -> Sum1/1
  Product3/1 -> Sum1/2
  Bias1/1 -> Direct Lookup Table (n-D)2/1
  In2/1 -> Direct Lookup Table (n-D)3/2, Direct Lookup Table (n-D)2/2
  Fcn1/1 -> Product3/2

== system rd3_mimo_sim_max/Plant/Actuators ==
  Comand : Inport
  coupled : Inport  Port=2
  Add : Sum  Inputs=3
  Gain1 : Gain  Gain=Bact  Multiplication=Matrix(K*u)
  Gain2 : Gain  Gain=Aact  Multiplication=Matrix(K*u)
  Gain3 : Gain  Gain=Bact_x  Multiplication=Matrix(K*u)
  Gain4 : Gain  Gain=Cact  Multiplication=Matrix(K*u)
  Gain5 : Gain  Gain=Cact_dot  Multiplication=Matrix(K*u)
  Integrator1 : Integrator
  Mux : Mux  Inputs=2
  To Workspace13 : ToWorkspace  VariableName=u_red_dot  SampleTime=-1
      settings: Decimation=data_deci
  Control : Outport
  States : Outport  Port=2
  wires:
  Gain1/1 -> Add/1
  Add/1 -> Integrator1/1
  Gain2/1 -> Add/2
  Integrator1/1 -> Gain4/1, Gain5/1, Gain2/1
  Comand/1 -> Gain1/1
  coupled/1 -> Gain3/1
  Gain3/1 -> Add/3
  Gain4/1 -> Control/1, Mux/1
  Gain5/1 -> Mux/2, To Workspace13/1
  Mux/1 -> States/1

== system rd3_mimo_sim_max/Plant/NonLinear VFA Model ==
  Controls : Inport
  Gust : Inport  Port=2
  Add1 : Sum  Inputs=+-
  Constant1 : Constant  Value=i_input_sel
  Constant3 : Constant  Value=6
  Constant5 : Constant  Value=i_state_sel
  Constant6 : Constant  Value=i_input_sel
  InputHold : Subsystem
  Mux2 : Mux  Inputs=2
  S-Function : S-Function  FunctionName=VFA_v1  Parameters=data,initstate  SFunctionDeploymentMode=off  EnableBusSupport=off
  Selector1 : Selector  InputPortWidth=size(Bp,2)  IndexOptions=Index vector (port)  Indices=[1 3]  OutputSizes=1
  Selector2 : Selector  InputPortWidth=length(Apsim)  IndexOptions=Index vector (port)  Indices=[1 3]  OutputSizes=1
  Selector3 : Selector  InputPortWidth=length(Apsim)  IndexOptions=Index vector (port)  Indices=[1 3]  OutputSizes=1
  Selector6 : Selector  InputPortWidth=size(Bp,2)  IndexOptions=Index vector (port)  Indices=[1 3]  OutputSizes=1
  StateHold : Subsystem
  Sum1 : Sum  Inputs=++|
  To Workspace1 : ToWorkspace  VariableName=d_red  SampleTime=-1
      settings: Decimation=data_deci
  To Workspace2 : ToWorkspace  VariableName=u_red  SampleTime=-1
      settings: Decimation=data_deci
  To Workspace4 : ToWorkspace  VariableName=u_red_hold  SampleTime=-1
      settings: Decimation=data_deci
  States : Outport
  States Rel. to Trim : Outport  Port=2
  eta : Outport  Port=3
  wires:
  Gust/1 -> To Workspace1/1, Mux2/2
  Mux2/1 -> S-Function/1
  Controls/1 -> Sum1/2
  Sum1/1 -> Selector1/1, Mux2/1
  Selector2/1 -> Add1/1, States/1
  Constant5/1 -> Selector2/2
  S-Function/1 -> Selector3/1, Selector2/1
  Constant1/1 -> Selector1/2
  Selector1/1 -> To Workspace2/1
  Constant3/1 -> Selector3/2
  Selector3/1 -> eta/1
  InputHold/1(u_trim) -> Sum1/1, Selector6/1
  Constant6/1 -> Selector6/2
  Selector6/1 -> To Workspace4/1
  StateHold/1(x_trim) -> Add1/2
  Add1/1 -> States Rel. to Trim/1

== system rd3_mimo_sim_max/Plant/Wind Gust Model ==
  Band-Limited White Noise : simulink/Sources/Band-Limited White Noise  Cov=tpower  Ts=samplet  seed=[23341]
  Band-Limited White Noise1 : simulink/Sources/Band-Limited White Noise  Cov=tpower  Ts=samplet  seed=[23342]
  Band-Limited White Noise2 : simulink/Sources/Band-Limited White Noise  Cov=tpower  Ts=samplet  seed=[23345]
  Band-Limited White Noise3 : simulink/Sources/Band-Limited White Noise  Cov=tpower  Ts=samplet  seed=[23361]
  Mux5 : Mux
  Gust : Outport
  wires:
  Band-Limited White Noise/1 -> Mux5/1
  Band-Limited White Noise1/1 -> Mux5/2
  Band-Limited White Noise2/1 -> Mux5/3
  Band-Limited White Noise3/1 -> Mux5/4
  Mux5/1 -> Gust/1

== system rd3_mimo_sim_max/Reference Model/Ahold ==
  State : Inport
  eta : Inport  Port=2
  Constant2 : Constant  Value=Aa_M
  Gain : Gain  Gain=180/pi
  Matrix Multiply6 : Product  Multiplication=Matrix(*)
  Subsystem1 : Subsystem
      mask Display: disp('matrix-interp');
  Out1 : Outport
  wires:
  eta/1 -> Gain/1
  Gain/1 -> Subsystem1/1(In1)
  Subsystem1/1(Out1) -> Matrix Multiply6/1
  State/1 -> Matrix Multiply6/2
  Matrix Multiply6/1 -> Out1/1
  Constant2/1 -> Subsystem1/2(In2)

== system rd3_mimo_sim_max/Adaptive Control/FL_Calculation/Filter1 ==
  u1 : Inport
  u1dot : Inport  Port=2
  u2 : Inport  Port=3
  u2dot : Inport  Port=4
  eta : Inport  Port=5
  Ba32_aug_hold : Subsystem
  Ba3_aug_hold1 : Subsystem
  Filter15 : Subsystem
      mask Display: disp('D1 Mixer')
  Gain10 : Gain  Gain=a20
  Matrix Multiply7 : Product  Multiplication=Matrix(*)
  Sum4 : Sum  Inputs=++|
  Out1 : Outport
  wires:
  u1/1 -> Matrix Multiply7/1, Filter15/1(u1)
  u1dot/1 -> Filter15/2(u1dot)
  u2/1 -> Matrix Multiply7/2, Filter15/3(u2)
  u2dot/1 -> Filter15/4(u2dot)
  Filter15/1(Out1) -> Ba32_aug_hold/1(State)
  Matrix Multiply7/1 -> Gain10/1
  Gain10/1 -> Ba3_aug_hold1/1(State)
  Ba32_aug_hold/1(Out1) -> Sum4/1
  Ba3_aug_hold1/1(Out1) -> Sum4/2
  Sum4/1 -> Out1/1
  eta/1 -> Ba3_aug_hold1/2(eta), Ba32_aug_hold/2(eta)

== system rd3_mimo_sim_max/Adaptive Control/FL_Calculation/Filter12 ==
  In1 : Inport
  Gain1 : Gain  Gain=a21/a22
  Gain10 : Gain  Gain=1/a22
  Gain2 : Gain  Gain=a20/a22
  Gain3 : Gain  Gain=a21
  Gain4 : Gain  Gain=a21
  Gain{5..9} (5 alike) : Gain  Gain=a22
  Integrator : Integrator
  Integrator1 : Integrator
  Sum : Sum  Inputs=|+--
  Sum1 : Sum  Inputs=|++
  Sum2 : Sum  Inputs=|++
  pi20 filter : Outport
  pi20 filter dot : Outport  Port=2
  pi20 filter ddot : Outport  Port=3
  pi21 filter : Outport  Port=4
  pi21 filter dot : Outport  Port=5
  wires:
  Integrator/1 -> Gain1/1, Gain6/1, Integrator1/1, Gain9/1, Gain4/1  "out_dot"
  Sum/1 -> Gain7/1, Integrator/1, Gain8/1  "out_ddot"
  Gain1/1 -> Sum/3
  Gain2/1 -> Sum/2
  Integrator1/1 -> Gain5/1, Gain3/1, Gain2/1  "out"
  Sum1/1 -> pi21 filter/1
  Gain3/1 -> Sum1/1
  Gain4/1 -> Sum2/1
  Sum2/1 -> pi21 filter dot/1
  Gain5/1 -> pi20 filter/1
  Gain6/1 -> pi20 filter dot/1
  Gain7/1 -> pi20 filter ddot/1
  Gain8/1 -> Sum2/2
  Gain9/1 -> Sum1/2
  In1/1 -> Gain10/1
  Gain10/1 -> Sum/1

== system rd3_mimo_sim_max/Adaptive Control/FL_Calculation/Filter13 ==
  u1 : Inport
  u1dot : Inport  Port=2
  u2 : Inport  Port=3
  u2dot : Inport  Port=4
  Gain2 : Gain  Gain=d10
  Gain25 : Gain  Gain=d11
  Matrix Multiply2 : Product  Multiplication=Matrix(*)
  Matrix Multiply3 : Product  Multiplication=Matrix(*)
  Sum2 : Sum  Inputs=++|
  Out1 : Outport
  wires:
  Matrix Multiply2/1 -> Gain2/1
  Matrix Multiply3/1 -> Gain25/1
  Gain25/1 -> Sum2/1
  u1dot/1 -> Matrix Multiply3/1
  u2/1 -> Matrix Multiply3/2
  u1/1 -> Matrix Multiply2/1
  u2dot/1 -> Matrix Multiply2/2
  Gain2/1 -> Sum2/2
  Sum2/1 -> Out1/1

== system rd3_mimo_sim_max/Adaptive Control/FL_Calculation/Filter2 ==
  u1 : Inport
  u1dot : Inport  Port=2
  u1ddot : Inport  Port=3
  u2 : Inport  Port=4
  u2dot : Inport  Port=5
  u2ddot : Inport  Port=6
  eta : Inport  Port=7
  Ba3_aug_hold1 : Subsystem
  Filter1 : Subsystem
      mask Display: disp('pi22 Mixer')
  Out1 : Outport
  wires:
  u2/1 -> Filter1/4(u2)
  u1/1 -> Filter1/1(u1)
  u1dot/1 -> Filter1/2(u1dot)
  u1ddot/1 -> Filter1/3(u1ddot)
  u2dot/1 -> Filter1/5(u2dot)
  u2ddot/1 -> Filter1/6(u2ddot)
  Filter1/1(Out1) -> Ba3_aug_hold1/1(State)
  Ba3_aug_hold1/1(Out1) -> Out1/1
  eta/1 -> Ba3_aug_hold1/2(eta)

== system rd3_mimo_sim_max/Adaptive Control/FL_Calculation/Filter3 ==
  u1 : Inport
  u1dot : Inport  Port=2
  u1ddot : Inport  Port=3
  u2 : Inport  Port=4
  u2dot : Inport  Port=5
  u2ddot : Inport  Port=6
  eta : Inport  Port=7
  Ba3_aug_hold1 : Subsystem
  Filter1 : Subsystem
      mask Display: disp('pi22 Mixer')
  Out1 : Outport
  wires:
  u2/1 -> Filter1/4(u2)
  u1/1 -> Filter1/1(u1)
  u1dot/1 -> Filter1/2(u1dot)
  u1ddot/1 -> Filter1/3(u1ddot)
  u2dot/1 -> Filter1/5(u2dot)
  u2ddot/1 -> Filter1/6(u2ddot)
  Filter1/1(Out1) -> Ba3_aug_hold1/1(State)
  Ba3_aug_hold1/1(Out1) -> Out1/1
  eta/1 -> Ba3_aug_hold1/2(eta)

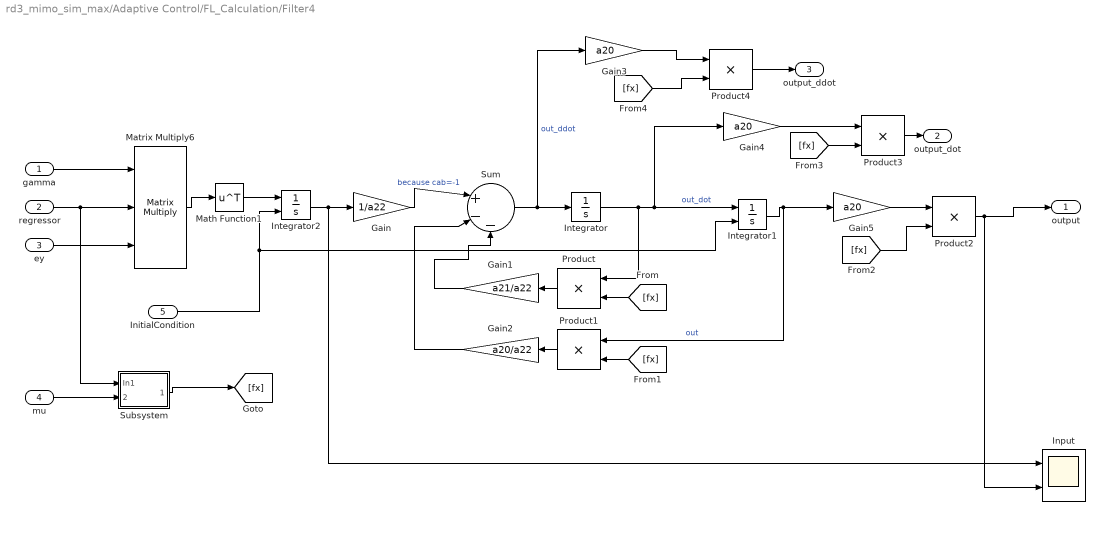
== system rd3_mimo_sim_max/Adaptive Control/FL_Calculation/Filter4 ==
  gamma : Inport
  regressor : Inport  Port=2
  ey : Inport  Port=3
  mu : Inport  Port=4
  InitialCondition : Inport  Port=5
  Gain : Gain  Gain=1/a22
  Gain1 : Gain  Gain=a21/a22
  Gain2 : Gain  Gain=a20/a22
  Gain3 : Gain  Gain=a20
  Gain4 : Gain  Gain=a20
  Gain5 : Gain  Gain=a20
  Input : Scope  NumInputPorts=2
  Integrator : Integrator
  Integrator1 : Integrator  InitialConditionSource=external  InitialCondition=lambda_0'
  Integrator2 : Integrator  InitialConditionSource=external  InitialCondition=lambda_0'
  Math Function1 : Math  Operator=transpose  SaturateOnIntegerOverflow=on
  Matrix Multiply6 : Product  Inputs=3  Multiplication=Matrix(*)
  Product{,1..4} (5 alike) : Product  RndMeth=Zero
  Subsystem : Subsystem
      mask Display: disp('f(x)');
  Sum : Sum  Inputs=|+--
  output : Outport
  output_dot : Outport  Port=2
  output_ddot : Outport  Port=3
  wires:
  Integrator/1 -> Product/1, Gain4/1, Integrator1/1  "out_dot"
  Sum/1 -> Integrator/1, Gain3/1  "out_ddot"
  Gain/1 -> Sum/1  "because cab=-1"
  Gain1/1 -> Sum/3
  Gain2/1 -> Sum/2
  Integrator1/1 -> Product1/1, Gain5/1  "out"
  gamma/1 -> Matrix Multiply6/1
  regressor/1 -> Subsystem/1(In1), Matrix Multiply6/2
  ey/1 -> Matrix Multiply6/3
  Subsystem/1(Out1) -> [fx]
  Product/1 -> Gain1/1
  [fx] -> Product/2
  Product1/1 -> Gain2/1
  [fx] -> Product1/2
  Integrator2/1 -> Input/1, Gain/1
  Gain5/1 -> Product2/1
  [fx] -> Product2/2
  Product2/1 -> Input/2, output/1
  Gain4/1 -> Product3/1
  Product3/1 -> output_dot/1
  [fx] -> Product3/2
  [fx] -> Product4/2
  Gain3/1 -> Product4/1
  Product4/1 -> output_ddot/1
  Matrix Multiply6/1 -> Math Function1/1
  Math Function1/1 -> Integrator2/1
  InitialCondition/1 -> Integrator1/2, Integrator2/2
  mu/1 -> Subsystem/2(mu_psi)

== system rd3_mimo_sim_max/Adaptive Control/FL_Calculation/Filter5 ==
  In1 : Inport
  Gain1 : Gain  Gain=a21/a22
  Gain10 : Gain  Gain=1/a22
  Gain2 : Gain  Gain=a20/a22
  Gain3 : Gain  Gain=a21
  Gain4 : Gain  Gain=a21
  Gain{5..9} (5 alike) : Gain  Gain=a22
  Integrator : Integrator
  Integrator1 : Integrator
  Sum : Sum  Inputs=|+--
  Sum1 : Sum  Inputs=|++
  Sum2 : Sum  Inputs=|++
  pi20 filter : Outport
  pi20 filter dot : Outport  Port=2
  pi20 filter ddot : Outport  Port=3
  pi21 filter : Outport  Port=4
  pi21 filter dot : Outport  Port=5
  wires:
  Integrator/1 -> Gain1/1, Gain6/1, Integrator1/1, Gain9/1, Gain4/1  "out_dot"
  Sum/1 -> Gain7/1, Integrator/1, Gain8/1  "out_ddot"
  Gain1/1 -> Sum/3
  Gain2/1 -> Sum/2
  Integrator1/1 -> Gain5/1, Gain3/1, Gain2/1  "out"
  Sum1/1 -> pi21 filter/1
  Gain3/1 -> Sum1/1
  Gain4/1 -> Sum2/1
  Sum2/1 -> pi21 filter dot/1
  Gain5/1 -> pi20 filter/1
  Gain6/1 -> pi20 filter dot/1
  Gain7/1 -> pi20 filter ddot/1
  Gain8/1 -> Sum2/2
  Gain9/1 -> Sum1/2
  In1/1 -> Gain10/1
  Gain10/1 -> Sum/1

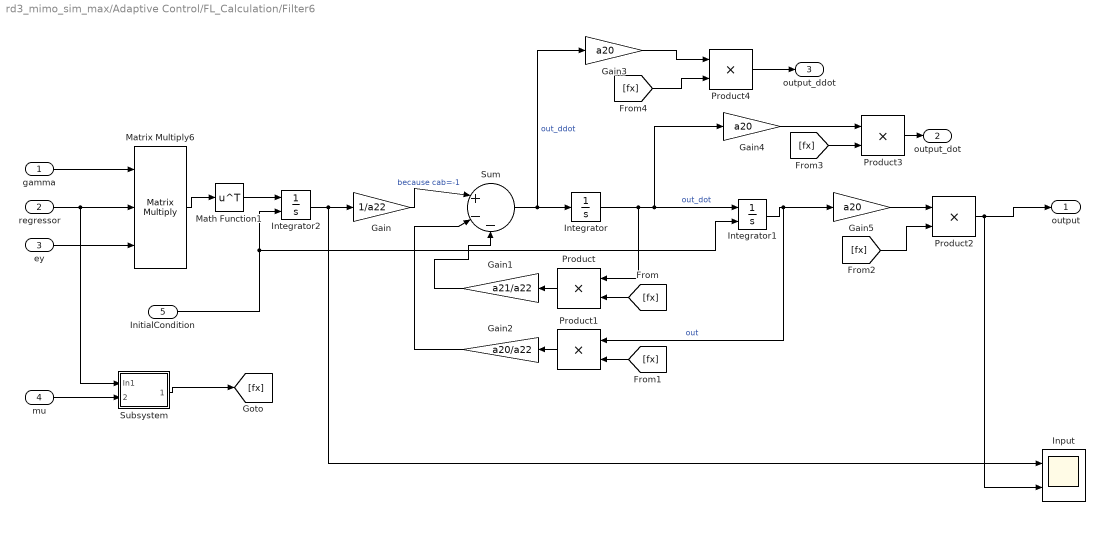
== system rd3_mimo_sim_max/Adaptive Control/FL_Calculation/Filter6 ==
  gamma : Inport
  regressor : Inport  Port=2
  ey : Inport  Port=3
  mu : Inport  Port=4
  InitialCondition : Inport  Port=5
  Gain : Gain  Gain=1/a22
  Gain1 : Gain  Gain=a21/a22
  Gain2 : Gain  Gain=a20/a22
  Gain3 : Gain  Gain=a20
  Gain4 : Gain  Gain=a20
  Gain5 : Gain  Gain=a20
  Input : Scope  NumInputPorts=2
  Integrator : Integrator
  Integrator1 : Integrator  InitialConditionSource=external  InitialCondition=lambda_0'
  Integrator2 : Integrator  InitialConditionSource=external  InitialCondition=lambda_0'
  Math Function1 : Math  Operator=transpose  SaturateOnIntegerOverflow=on
  Matrix Multiply6 : Product  Inputs=3  Multiplication=Matrix(*)
  Product{,1..4} (5 alike) : Product  RndMeth=Zero
  Subsystem : Subsystem
      mask Display: disp('f(x)');
  Sum : Sum  Inputs=|+--
  output : Outport
  output_dot : Outport  Port=2
  output_ddot : Outport  Port=3
  wires:
  Integrator/1 -> Product/1, Gain4/1, Integrator1/1  "out_dot"
  Sum/1 -> Integrator/1, Gain3/1  "out_ddot"
  Gain/1 -> Sum/1  "because cab=-1"
  Gain1/1 -> Sum/3
  Gain2/1 -> Sum/2
  Integrator1/1 -> Product1/1, Gain5/1  "out"
  gamma/1 -> Matrix Multiply6/1
  regressor/1 -> Subsystem/1(In1), Matrix Multiply6/2
  ey/1 -> Matrix Multiply6/3
  Subsystem/1(Out1) -> [fx]
  Product/1 -> Gain1/1
  [fx] -> Product/2
  Product1/1 -> Gain2/1
  [fx] -> Product1/2
  Integrator2/1 -> Input/1, Gain/1
  Gain5/1 -> Product2/1
  [fx] -> Product2/2
  Product2/1 -> Input/2, output/1
  Gain4/1 -> Product3/1
  Product3/1 -> output_dot/1
  [fx] -> Product3/2
  [fx] -> Product4/2
  Gain3/1 -> Product4/1
  Product4/1 -> output_ddot/1
  Matrix Multiply6/1 -> Math Function1/1
  Math Function1/1 -> Integrator2/1
  InitialCondition/1 -> Integrator1/2, Integrator2/2
  mu/1 -> Subsystem/2(mu_psi)

== system rd3_mimo_sim_max/Adaptive Control/Fxm_Calculation/Filter1 ==
  u1 : Inport
  u1dot : Inport  Port=2
  u2 : Inport  Port=3
  u2dot : Inport  Port=4
  eta : Inport  Port=5
  Ba32_hold : Subsystem
  Ba3_hold1 : Subsystem
  Filter15 : Subsystem
      mask Display: disp('D1 Mixer')
  Gain10 : Gain  Gain=a20
  Matrix Multiply7 : Product  Multiplication=Matrix(*)
  Sum4 : Sum  Inputs=++|
  Out1 : Outport
  wires:
  u1/1 -> Matrix Multiply7/1, Filter15/1(u1)
  u1dot/1 -> Filter15/2(u1dot)
  u2/1 -> Matrix Multiply7/2, Filter15/3(u2)
  u2dot/1 -> Filter15/4(u2dot)
  Filter15/1(Out1) -> Ba32_hold/1(State)
  Matrix Multiply7/1 -> Gain10/1
  Gain10/1 -> Ba3_hold1/1(State)
  Ba32_hold/1(Out1) -> Sum4/1
  Ba3_hold1/1(Out1) -> Sum4/2
  Sum4/1 -> Out1/1
  eta/1 -> Ba3_hold1/2(eta), Ba32_hold/2(eta)

== system rd3_mimo_sim_max/Adaptive Control/Fxm_Calculation/Filter12 ==
  In1 : Inport
  Gain1 : Gain  Gain=a21/a22
  Gain10 : Gain  Gain=1/a22
  Gain2 : Gain  Gain=a20/a22
  Gain3 : Gain  Gain=a21
  Gain4 : Gain  Gain=a21
  Gain{5..9} (5 alike) : Gain  Gain=a22
  Integrator : Integrator
  Integrator1 : Integrator
  Sum : Sum  Inputs=|+--
  Sum1 : Sum  Inputs=|++
  Sum2 : Sum  Inputs=|++
  pi20 filter : Outport
  pi20 filter dot : Outport  Port=2
  pi20 filter ddot : Outport  Port=3
  pi21 filter : Outport  Port=4
  pi21 filter dot : Outport  Port=5
  wires:
  Integrator/1 -> Gain1/1, Gain6/1, Integrator1/1, Gain9/1, Gain4/1  "out_dot"
  Sum/1 -> Gain7/1, Integrator/1, Gain8/1  "out_ddot"
  Gain1/1 -> Sum/3
  Gain2/1 -> Sum/2
  Integrator1/1 -> Gain5/1, Gain3/1, Gain2/1  "out"
  Sum1/1 -> pi21 filter/1
  Gain3/1 -> Sum1/1
  Gain4/1 -> Sum2/1
  Sum2/1 -> pi21 filter dot/1
  Gain5/1 -> pi20 filter/1
  Gain6/1 -> pi20 filter dot/1
  Gain7/1 -> pi20 filter ddot/1
  Gain8/1 -> Sum2/2
  Gain9/1 -> Sum1/2
  In1/1 -> Gain10/1
  Gain10/1 -> Sum/1

== system rd3_mimo_sim_max/Adaptive Control/Fxm_Calculation/Filter13 ==
  u1 : Inport
  u1dot : Inport  Port=2
  u2 : Inport  Port=3
  u2dot : Inport  Port=4
  Gain2 : Gain  Gain=d10
  Gain25 : Gain  Gain=d11
  Matrix Multiply2 : Product  Multiplication=Matrix(*)
  Matrix Multiply3 : Product  Multiplication=Matrix(*)
  Sum2 : Sum  Inputs=++|
  Out1 : Outport
  wires:
  Matrix Multiply2/1 -> Gain2/1
  Matrix Multiply3/1 -> Gain25/1
  Gain25/1 -> Sum2/1
  u1dot/1 -> Matrix Multiply3/1
  u2/1 -> Matrix Multiply3/2
  u1/1 -> Matrix Multiply2/1
  u2dot/1 -> Matrix Multiply2/2
  Gain2/1 -> Sum2/2
  Sum2/1 -> Out1/1

== system rd3_mimo_sim_max/Adaptive Control/Fxm_Calculation/Filter2 ==
  u1 : Inport
  u1dot : Inport  Port=2
  u2 : Inport  Port=3
  u2dot : Inport  Port=4
  Gain2 : Gain  Gain=d10
  Gain25 : Gain  Gain=d11
  Matrix Multiply2 : Product  Multiplication=Matrix(*)
  Matrix Multiply3 : Product  Multiplication=Matrix(*)
  Sum2 : Sum  Inputs=++|
  Out1 : Outport
  wires:
  Matrix Multiply2/1 -> Gain2/1
  Matrix Multiply3/1 -> Gain25/1
  Gain25/1 -> Sum2/1
  u1dot/1 -> Matrix Multiply3/1
  u2/1 -> Matrix Multiply3/2
  u1/1 -> Matrix Multiply2/1
  u2dot/1 -> Matrix Multiply2/2
  Gain2/1 -> Sum2/2
  Sum2/1 -> Out1/1

== system rd3_mimo_sim_max/Adaptive Control/Fxm_Calculation/Filter3 ==
  u1 : Inport
  u1dot : Inport  Port=2
  u1ddot : Inport  Port=3
  u2 : Inport  Port=4
  u2dot : Inport  Port=5
  u2ddot : Inport  Port=6
  eta : Inport  Port=7
  Ba3_hold1 : Subsystem
  Filter1 : Subsystem
      mask Display: disp('pi22 Mixer')
  Out1 : Outport
  wires:
  u2/1 -> Filter1/4(u2)
  u1/1 -> Filter1/1(u1)
  u1dot/1 -> Filter1/2(u1dot)
  u1ddot/1 -> Filter1/3(u1ddot)
  u2dot/1 -> Filter1/5(u2dot)
  u2ddot/1 -> Filter1/6(u2ddot)
  Filter1/1(Out1) -> Ba3_hold1/1(State)
  Ba3_hold1/1(Out1) -> Out1/1
  eta/1 -> Ba3_hold1/2(eta)

== system rd3_mimo_sim_max/Adaptive Control/Fxm_Calculation/Filter4 ==
  In1 : Inport
  Gain1 : Gain  Gain=a21/a22
  Gain10 : Gain  Gain=1/a22
  Gain2 : Gain  Gain=a20/a22
  Gain3 : Gain  Gain=a21
  Gain4 : Gain  Gain=a21
  Gain{5..9} (5 alike) : Gain  Gain=a22
  Integrator : Integrator
  Integrator1 : Integrator
  Sum : Sum  Inputs=|+--
  Sum1 : Sum  Inputs=|++
  Sum2 : Sum  Inputs=|++
  pi20 filter : Outport
  pi20 filter dot : Outport  Port=2
  pi20 filter ddot : Outport  Port=3
  pi21 filter : Outport  Port=4
  pi21 filter dot : Outport  Port=5
  wires:
  Integrator/1 -> Gain1/1, Gain6/1, Integrator1/1, Gain9/1, Gain4/1  "out_dot"
  Sum/1 -> Gain7/1, Integrator/1, Gain8/1  "out_ddot"
  Gain1/1 -> Sum/3
  Gain2/1 -> Sum/2
  Integrator1/1 -> Gain5/1, Gain3/1, Gain2/1  "out"
  Sum1/1 -> pi21 filter/1
  Gain3/1 -> Sum1/1
  Gain4/1 -> Sum2/1
  Sum2/1 -> pi21 filter dot/1
  Gain5/1 -> pi20 filter/1
  Gain6/1 -> pi20 filter dot/1
  Gain7/1 -> pi20 filter ddot/1
  Gain8/1 -> Sum2/2
  Gain9/1 -> Sum1/2
  In1/1 -> Gain10/1
  Gain10/1 -> Sum/1

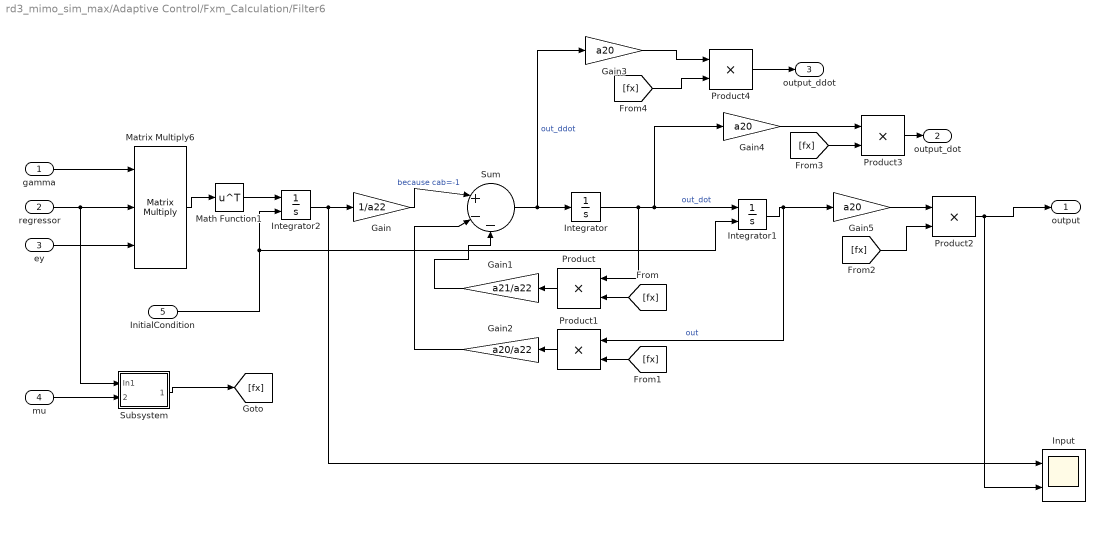
== system rd3_mimo_sim_max/Adaptive Control/Fxm_Calculation/Filter6 ==
  gamma : Inport
  regressor : Inport  Port=2
  ey : Inport  Port=3
  mu : Inport  Port=4
  InitialCondition : Inport  Port=5
  Gain : Gain  Gain=1/a22
  Gain1 : Gain  Gain=a21/a22
  Gain2 : Gain  Gain=a20/a22
  Gain3 : Gain  Gain=a20
  Gain4 : Gain  Gain=a20
  Gain5 : Gain  Gain=a20
  Input : Scope  NumInputPorts=2
  Integrator : Integrator
  Integrator1 : Integrator  InitialConditionSource=external  InitialCondition=lambda_0'
  Integrator2 : Integrator  InitialConditionSource=external  InitialCondition=lambda_0'
  Math Function1 : Math  Operator=transpose  SaturateOnIntegerOverflow=on
  Matrix Multiply6 : Product  Inputs=3  Multiplication=Matrix(*)
  Product{,1..4} (5 alike) : Product  RndMeth=Zero
  Subsystem : Subsystem
      mask Display: disp('f(x)');
  Sum : Sum  Inputs=|+--
  output : Outport
  output_dot : Outport  Port=2
  output_ddot : Outport  Port=3
  wires:
  Integrator/1 -> Product/1, Gain4/1, Integrator1/1  "out_dot"
  Sum/1 -> Integrator/1, Gain3/1  "out_ddot"
  Gain/1 -> Sum/1  "because cab=-1"
  Gain1/1 -> Sum/3
  Gain2/1 -> Sum/2
  Integrator1/1 -> Product1/1, Gain5/1  "out"
  gamma/1 -> Matrix Multiply6/1
  regressor/1 -> Subsystem/1(In1), Matrix Multiply6/2
  ey/1 -> Matrix Multiply6/3
  Subsystem/1(Out1) -> [fx]
  Product/1 -> Gain1/1
  [fx] -> Product/2
  Product1/1 -> Gain2/1
  [fx] -> Product1/2
  Integrator2/1 -> Input/1, Gain/1
  Gain5/1 -> Product2/1
  [fx] -> Product2/2
  Product2/1 -> Input/2, output/1
  Gain4/1 -> Product3/1
  Product3/1 -> output_dot/1
  [fx] -> Product3/2
  [fx] -> Product4/2
  Gain3/1 -> Product4/1
  Product4/1 -> output_ddot/1
  Matrix Multiply6/1 -> Math Function1/1
  Math Function1/1 -> Integrator2/1
  InitialCondition/1 -> Integrator1/2, Integrator2/2
  mu/1 -> Subsystem/2(mu_psi)

== system rd3_mimo_sim_max/Adaptive Control/S1hold/Subsystem1 ==
  In1 : Inport
  In2 : Inport  Port=2
  Bias1 : Bias  Bias=1
  Direct Lookup Table (n-D)2 : LookupNDDirect  NumberOfTableDimensions=3  InputsSelectThisObjectFromTable=2-D Matrix  TableIsInput=on  Table=ahold
  Direct Lookup Table (n-D)3 : LookupNDDirect  NumberOfTableDimensions=3  InputsSelectThisObjectFromTable=2-D Matrix  TableIsInput=on  Table=ahold
  Fcn1 : Fcn  Expr=1-u(1)
  Prelookup1 : PreLookup  BreakpointsData=etasweep  ExtrapMethod=Linear
  Product2 : Product  RndMeth=Zero
  Product3 : Product  RndMeth=Zero
  Sum1 : Sum  Inputs=|++
  Out1 : Outport
  wires:
  In1/1 -> Prelookup1/1
  Sum1/1 -> Out1/1
  Prelookup1/1 -> Direct Lookup Table (n-D)3/1, Bias1/1
  Direct Lookup Table (n-D)2/1 -> Product2/1
  Prelookup1/2 -> Product2/2, Fcn1/1
  Direct Lookup Table (n-D)3/1 -> Product3/1
  Product2/1 -> Sum1/1
  Product3/1 -> Sum1/2
  Bias1/1 -> Direct Lookup Table (n-D)2/1
  In2/1 -> Direct Lookup Table (n-D)3/2, Direct Lookup Table (n-D)2/2
  Fcn1/1 -> Product3/2
